simulink model "danlianganbihuan"  (R2025b)
settings: Solver=VariableStepAuto  StartTime=0.0  StopTime=10.0  RelTol=1e-3
settings Model: Creator=allen  LastModifiedBy=allen

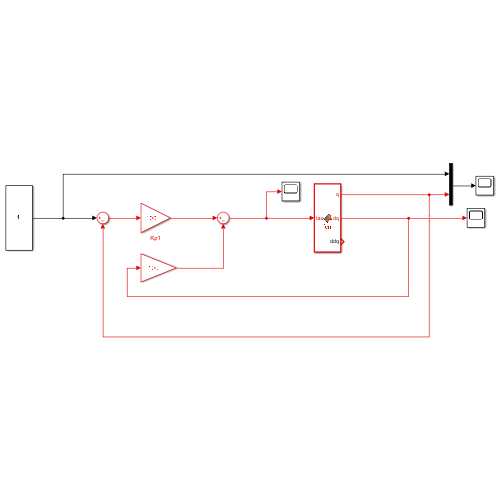
[thumbnail: Simulink's stored preview of the top-level diagram]
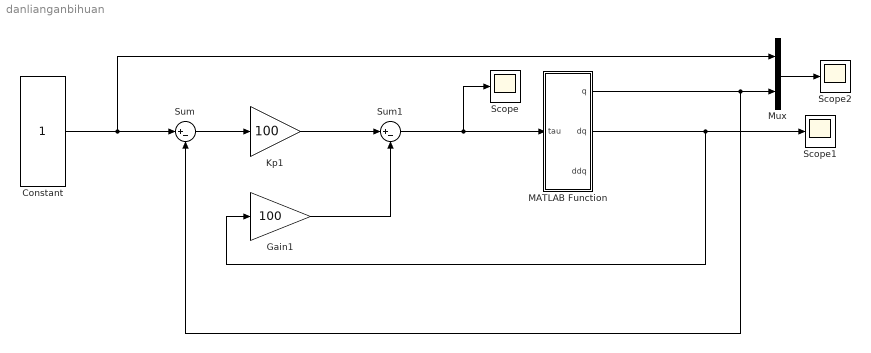
== system danlianganbihuan ==
  Constant : Constant
  Gain1 : Gain  Gain=100
  Kp1 : Gain  Gain=100
  MATLAB Function : MATLAB Function  TreatAsAtomicUnit=on
  Mux : Mux  Inputs=2
  Scope : Scope
  Scope1 : Scope
  Scope2 : Scope
      settings: DataLoggingVariableName=ScopeData2
  Sum : Sum  Inputs=|+-
  Sum1 : Sum  Inputs=|+-
  wires:
  Constant/1 -> Mux/1, Sum/1
  Sum/1 -> Kp1/1
  Kp1/1 -> Sum1/1
  Gain1/1 -> Sum1/2
  Sum1/1 -> Scope/1, MATLAB Function/1(tau)
  MATLAB Function/2(dq) -> Gain1/1, Scope1/1
  Mux/1 -> Scope2/1
  MATLAB Function/1(q) -> Sum/2, Mux/2

== matlab function danlianganbihuan/MATLAB Function ==
  data: tau input; q output; dq output; ddq output
function [q, dq, ddq] = fcn(tau)

persistent q_k dq_k
if isempty(q_k)
    q_k = 0;
end
if isempty(dq_k)
    dq_k = 0;
end

H = 0.0833;
ddq = tau / H;

Ts = 0.001;
q_k = q_k + dq_k * Ts;
dq_k = dq_k + ddq * Ts;

q = q_k;
dq = dq_k;
end
